simulink subsystem "Day2_Scenario_2_3"  (R2024a)
settings: Solver=VariableStepAuto  StartTime=0.0  StopTime=10.0  RelTol=1e-3
libraries: CarMaker4SL x6
settings Model: Creator=junhyung.cha  LastModifiedBy=pc

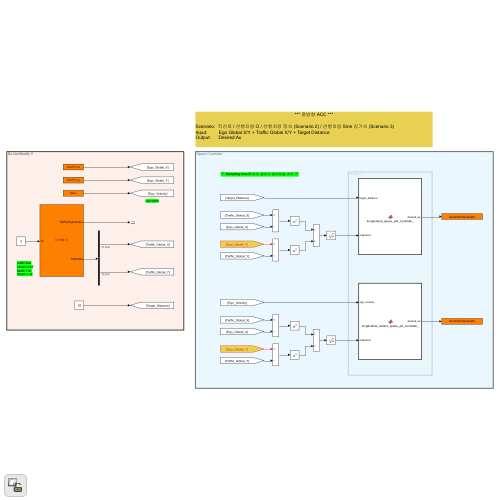
[thumbnail: Simulink's stored preview of the top-level diagram]
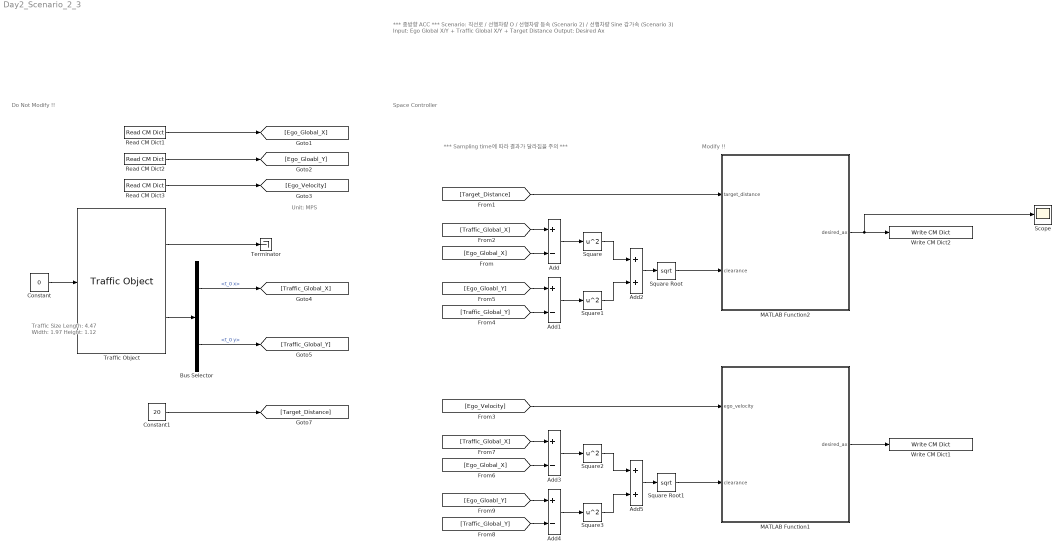
== system Day2_Scenario_2_3 ==
  note: *** Sampling time에 따라 결과가 달라짐을 주의 ***
  note: Space Controller
  note: Modify !!
  note: Do Not Modify !!
  note: Traffic Size
      | Length: 4.47
      | Width: 1.97
      | Height: 1.12
  note: *** 종방향 ACC ***
      |
      | Scenario: 직선로 / 선행차량 O / 선행차량 등속 (Scenario 2) / 선행차량 Sine 감가속 (Scenario 3)
      | Input: Ego Global X/Y + Traffic Global X/Y + Target Distance
      | Output: Desired Ax
  note: Unit: MPS
  Add{,1,3..4} (4 alike) : Sum  Inputs=+-
  Add2 : Sum
  Add5 : Sum
  Bus Selector : BusSelector  OutputSignals=t_0 x,t_0 y
  Constant : Constant  Value=0
  Constant1 : Constant  Value=20
  MATLAB Function1 : MATLAB Function  TreatAsAtomicUnit=on
  MATLAB Function2 : MATLAB Function  TreatAsAtomicUnit=on
  Read CM Dict1 : CarMaker4SL/Read CM Dict  xname=Car.Fr1.tx  xsync=off  xstime=Inherited
  Read CM Dict2 : CarMaker4SL/Read CM Dict  xname=Car.Fr1.ty  xsync=off  xstime=Inherited
  Read CM Dict3 : CarMaker4SL/Read CM Dict  xname=Car.v  xsync=off  xstime=Inherited
  Scope : Scope
  Square{,1..3} (4 alike) : Math  Operator=square
  Square Root : Sqrt
  Square Root1 : Sqrt
  Terminator : Terminator
  Traffic Object : CarMaker4SL/Traffic Object  xname=T00  ximode=Traffic Id  xstime=Inherited
      settings: SourceProductName=CarMaker4SL
  Write CM Dict1 : CarMaker4SL/Write CM Dict  xname=AccelCtrl.DesiredAx  xsync=off
  Write CM Dict2 : CarMaker4SL/Write CM Dict  xname=AccelCtrl.DesiredAx  xsync=off
  wires:
  Read CM Dict2/1 -> [Ego_Gloabl_Y]
  MATLAB Function2/1(desired_ax) -> Write CM Dict2/1, Scope/1
  Read CM Dict1/1 -> [Ego_Global_X]
  Constant/1 -> Traffic Object/1
  Traffic Object/2 -> Bus Selector/1
  Traffic Object/1 -> Terminator/1
  Bus Selector/1 -> [Traffic_Global_X]  "<t_0 x>"
  Bus Selector/2 -> [Traffic_Global_Y]  "<t_0 y>"
  Square Root/1 -> MATLAB Function2/2(clearance)
  Constant1/1 -> [Target_Distance]
  [Ego_Global_X] -> Add/2
  [Traffic_Global_X] -> Add/1
  [Traffic_Global_Y] -> Add1/2
  [Ego_Gloabl_Y] -> Add1/1
  Add1/1 -> Square1/1
  Add2/1 -> Square Root/1
  Square/1 -> Add2/1
  Square1/1 -> Add2/2
  [Target_Distance] -> MATLAB Function2/1(target_distance)
  Add/1 -> Square/1
  Read CM Dict3/1 -> [Ego_Velocity]
  [Ego_Velocity] -> MATLAB Function1/1(ego_velocity)
  Add3/1 -> Square2/1
  Square3/1 -> Add5/2
  Square2/1 -> Add5/1
  Add5/1 -> Square Root1/1
  Add4/1 -> Square3/1
  [Ego_Gloabl_Y] -> Add4/1
  [Traffic_Global_Y] -> Add4/2
  [Traffic_Global_X] -> Add3/1
  [Ego_Global_X] -> Add3/2
  Square Root1/1 -> MATLAB Function1/2(clearance)
  MATLAB Function1/1(desired_ax) -> Write CM Dict1/1

== matlab function Day2_Scenario_2_3/MATLAB Function1 ==
  settings: updateMethod=DISCRETE  sampleTime=0.05
  data: ego_velocity input; desired_ax output; clearance input
function desired_ax = longitudinal_space_pid_controller_(ego_velocity, clearance)
%#codegen
% longitudinal_space_pid_controller_  - Time–Gap Policy 적용 (입력 2개)
%
%  ego_velocity  : Ego 차량 속도 [m/s]
%  clearance     : 전방 차량과의 실제 간격 [m]
%  desired_ax    : 출력 가속도 명령   [m/s^2]

  %% --- 파라미터 및 상태 변수 초기화 ---
  persistent prev_error integral
  persistent Kp Ki Kd dt d0 time_gap
  if isempty(prev_error)
    dt       = 0.01;   % 샘플 시간 [s]
    Kp       = 0.12;   % 비례 게인
    Ki       = 0.008;  % 적분 게인
    Kd       = 0.225;  % 미분 게인

    d0       = 2.0;    % 최소 여유 거리 [m] (clearance 최소값)
    time_gap = 0.2;    % 설정 시간 헤드웨이 [s]

    prev_error = 0;
    integral   = 0;
  end

  %% 1) 목표 간격 계산 (Time–Gap Policy)
  desired_distance = d0 + ego_velocity * time_gap;

  %% 2) 에러 계산
  error = clearance - desired_distance;

  %% 3) PID 계산
  integral   = integral + error * dt;
  derivative = (error - prev_error) / dt;
  desired_ax = Kp * error + Ki * integral + Kd * derivative;

  %% 4) 상태 업데이트
  prev_error = error;
end

== matlab function Day2_Scenario_2_3/MATLAB Function2 ==
  settings: updateMethod=DISCRETE  sampleTime=0.05
  data: target_distance input; desired_ax output; clearance input
function desired_ax = longitudinal_space_pid_controller_(target_distance, clearance)
%#codegen
% target_distance : measured distance to lead vehicle [m]
% clearance       : desired spacing [m]
% desired_ax      : output acceleration command [m/s^2]

  %% persistent 변수 선언
  persistent prev_e integral
  persistent Kp Ki Kd dt
  if isempty(prev_e)
    % === 파라미터 초기화 (필요에 따라 수정) ===
    dt = 0.05;       % 샘플 시간 [s]
    Kp = 0.1;      % 비례 게인
    Ki = 0;     % 적분 게인
    Kd = 0.5;     % 미분 게인

    prev_e = 0;
    integral = 0;
  end

  %% 1) 오차 계산
  e = (clearance - target_distance);

  %% 2) 적분항 업데이트
  integral = integral + e * dt;

  %% 3) 미분항 계산
  deriv = (e - prev_e) / dt;

  %% 4) PID 합산
  desired_ax = Kp * e + Ki * integral + Kd * deriv;

  %% 5) 이전 오차 갱신
  prev_e = e;
end
